simulink model "callGAMS"  (R2021b)
settings: Solver=ode1  StartTime=0.0  StopTime=20  FixedStep=1e-4  RelTol=1e-3
model workspace (MAT data in the model file):
  firstOrder = 60
  g2Max = 0
  runTime = 4
undefined symbols (not defined in the file or in its folder): c0, c1, D11, Delta, fg, G2gen, G3gen, G5gen, G6gen, G7gen, Iovc, l0, l1, Newton, r0, r1, Raphson, Rtpu, S1non, S2non, S3non, S5non, S6non, S7non, sigbuilder_block, tonvsc, Ts, Vhv, Vmv, w_pll, wc1, wdc1, wpq1, wsw1, Xtpu
libraries: simulink_extras x122, simulink x73, spsFirstOrderFilterLib x72, spsGroundLib x61, spsCurrentMeasurementLib x33, spsVoltageMeasurementLib x33, eeTransforms x24, spsabctoAlphaBetaZeroLib x12, spsControlledVoltageSourceLib x12, spsControlledCurrentSourceLib x12, spsPower3phPhasorLib x11, spsLoadFlowBusLib x9
(part 2 of 16)

== system callGAMS/sm_computation/G2 ==
  Bus Selector : BusSelector  OutputSignals=Pabc,Qabc,vqp,vdp,vqn,vdn,iqp,idp,iqn,idn,f
  Constant1 : Constant  Value=5e6
  G2 setpoint : Subsystem
  Goto1 : Goto  Commented=on  GotoTag=Pg2  TagVisibility=global
  Goto3 : Goto  Commented=on  GotoTag=vdqpng2  TagVisibility=global
  Goto4 : Goto  Commented=on  GotoTag=idqpng2  TagVisibility=global
  Goto5 : Goto  Commented=on  GotoTag=Qg2  TagVisibility=global
  Mux2 : Mux
  Mux3 : Mux
  VSC v2 : Subsystem  mask{vscmod=Phasor I-ref, fg=fg, Vhv=Vhv, Vmv=Vmv, Pconv=S2non, Rtpu=Rtpu, Xtpu=Xtpu, qmode=Active power, dmode=Reactive power, wsw=wsw1, wn_pll=w_pll, wc=wc1, wpq=wpq1, wdc=wdc1, koc=Iovc, Cdc=3100e-6, tfilt=1*(1/wsw1), negseq_en=off, fdroop_en=on, Vacdroop_en=off, LVRT_en=off, Kfdroop=0.05, fdroop_per=10, Kvdroop=0.1, Vacdroop_per=10, Vlvrt0=0.9, Vlvrt_min=0.5, Qmax_lvrt=0.9, V0pu=0.99605, theta0=-30.4161, P0=S2non*G2gen, Q0=5e6}
      mask prompts: vscmod "VSC Model"; fg "AC grid frequency (Hz)"; Vhv "Grid-side voltage (V)(LL-rms)"; Vmv "Converter-side voltage (V)(LL-rms)"; Pconv "Converter nominal power (VA)"; Rtpu "Resistance seen by the converter (p.u)"; Xtpu "Reactance seen by the converter (p.u)"; qmode "q-axis control mode"; dmode "d-axis control mode"; wsw "Switching frequency (rad/s)"; wn_pll "PLL filter natural frequency"; wc "Current-control bandwidth (rad/s)"; wpq "PQ control bandwidth (rad/s)"; wdc "DC Voltage control bandwidth(rad/s)"; koc "Overcurrent factor (p.u)"; Cdc "DC-side total capacitance (F)"; tfilt "Vabc filter time constant (s)"; negseq_en "Enable negative sequence control"; fdroop_en "Enable frequency droop"; Vacdroop_en "Enable AC voltage droop"; LVRT_en "Enable LVRT"; Kfdroop "Frequency droop (p.u)"; fdroop_per "Percentage of converter power to contribute with droop (%)"; Kvdroop "Voltage droop (p.u)"; Vacdroop_per "Percentage of converter power to contribute with droop (%)"; Vlvrt0 "initial voltage (p.u)"; Vlvrt_min "minimum voltage (p.u)"; Qmax_lvrt "max power injected at min voltage (p.u)"; V0pu "Initial terminal voltage magnitude (pu)"; theta0 "Initial terminal voltage angle (deg)"; P0 "Initial active power (W)"; Q0 "Initial reactive power (VAr)"
      mask init:
      | %% ----------------------VSC Parameters-------------------------- %%
      | j = 1i;
      | r = Vhv/Vmv;                    % Transformer ratio
      | Vmvpk = Vmv*sqrt(2)/sqrt(3);    % Converter-side voltage phase-to-ground peak-to-peak
      | Vhvpk = Vhv*sqrt(2)/sqrt(3);    % Grid-side voltage phase-to-ground peak-to-peak  
      | Vdc = 2*Vhvpk;                  % Nominal DC voltage 
      | ksw = round(wsw/(2*pi*fg));      % Calculates switching ratio
      | Iconvbase = 2*Pconv/(3*Vmvpk);  % Converter base current (A)
      | Zbmv = Vmv^2/Pconv;             % Base voltage referred to the converter side
      | Imax = koc*Iconvbase;   % Converter maximum output current
      | %Cdc = 2*Hvsc*Pconv/Vdc^2;       % DC capacitor
      | 
      | Xt = Xtpu*Zbmv;        % p.u to (Ohms)
      | Lt = Xt/(2*pi*fg);              % p.u to (H)
      | Rt = Rtpu*Zbmv;        % p.u. to (Ohms)
      | 
      | % -------------LVRT--------------%
      | Klvrt = Qmax_lvrt/(Vlvrt_min-Vlvrt0); % Defines LVRT inclination of the V/I LVRT characteristic
      | 
      | % ------------ PLL ------------- %
      | zeta_pll = 1/sqrt(2);           % Damping
      | kp_pll = 2*zeta_pll*wn_pll/(Vmvpk);
      | tau_pll = 2*zeta_pll/wn_pll;
      | 
      | % ------------ Inner-loop (current control) ------------ %
      | kp_c = Lt*wc; 
      | ti_c = Lt/Rt;
      | 
      | % -------- Outer-loop (voltage and/or power control)
      | % --- PQ closed-loop control ----
      | ti_pq = 1/wc;
      | kp_pq = 2/3*ti_pq*wpq*1/Vmvpk;
      | 
      | % --- Vdc control ----
      | damp_dc = 1/sqrt(2);
      | kp_dc = 2*Cdc*damp_dc*wdc; 
      | ki_dc = Cdc*wdc^2;
      | 
      | %% ---------------------Mask operations----------------------------%%
      | 
      | % If the box is unchecked, we set the bias value to zero
      | if ~fdroop_en; end
      | if ~Vacdroop_en; end
      | if ~LVRT_en; Klvrt = 0;  end
      | 
      | %% -------------------- Variant Subsystem ----------------------- %%
      | choice = get_param(gcb,'vscmod'); % Get choice from list
      | VSS_model = [gcb, '/VSC Model'];  % VSC electrical Model
      | VSS_meas = [gcb, '/VSC Control/Measurements']; % Measurements (PLL, Park transformation, etc)
      | VSS_mod = [gcb, '/VSC Control/Modulation']; % Modulation or reference voltage/current generation
      | VSS_ctr = [gcb, '/VSC Control/Control loops']; % Modulation or reference voltage/current generation
      | 
      | 
      | if strcmp(choice,'EMT Switching')
      |     set_param(VSS_model, 'LabelModeActiveChoice', 'EMT_SW');
      |     set_param(VSS_meas, 'LabelModeActiveChoice', 'EMT');
      |     set_param(VSS_mod, 'LabelModeActiveChoice', 'EMT_SW');
      |     set_param(VSS_ctr, 'LabelModeActiveChoice', 'EMT_and_QEMT');
      |     
      | elseif strcmp(choice,'EMT Average')
      |     set_param(VSS_model, 'LabelModeActiveChoice', 'EMT_AVG');
      |     set_param(VSS_meas, 'LabelModeActiveChoice', 'EMT');
      |     set_param(VSS_mod, 'LabelModeActiveChoice', 'EMT_AVG');
      |     set_param(VSS_ctr, 'LabelModeActiveChoice', 'EMT_and_QEMT');
      |     %set_param([VSS_meas '/EMT/Vabc filter'],'Commented','through')
      |     tfilt = 0; % No filtering in Average model
      |     
      | elseif strcmp(choice,'Phasor Quasi-EMT')
      |     set_param(VSS_model, 'LabelModeActiveChoice', 'Phasor');
      |     set_param(VSS_meas, 'LabelModeActiveChoice', 'Phasor');
      |     set_param(VSS_mod, 'LabelModeActiveChoice', 'Phasor_QEMT');
      |     set_param(VSS_ctr, 'LabelModeActiveChoice', 'EMT_and_QEMT');
      |     
      | elseif strcmp(choice,'Phasor I-1st')
      |     set_param(VSS_model, 'LabelModeActiveChoice', 'Phasor');
      |     set_param(VSS_meas, 'LabelModeActiveChoice', 'Phasor');
      |     set_param(VSS_mod, 'LabelModeActiveChoice', 'Phasor_I_and_PQ');
      |     set_param(VSS_ctr, 'LabelModeActiveChoice', 'Phasor_I_1st');
      |     
      | elseif strcmp(choice,'Phasor I-ref')
      |     set_param(VSS_model, 'LabelModeActiveChoice', 'Phasor');
      | 	set_param(VSS_meas, 'LabelModeActiveChoice', 'Phasor');
      |     set_param(VSS_mod, 'LabelModeActiveChoice', 'Phasor_I_and_PQ');
      |     set_param(VSS_ctr, 'LabelModeActiveChoice', 'Phasor_I_ref');
      |     
      | elseif strcmp(choice,'Phasor PQ-1st')
      |     set_param(VSS_model, 'LabelModeActiveChoice', 'Phasor');
      |     set_param(VSS_meas, 'LabelModeActiveChoice', 'Phasor');
      |     set_param(VSS_mod, 'LabelModeActiveChoice', 'Phasor_I_and_PQ');
      |     set_param(VSS_ctr, 'LabelModeActiveChoice', 'Phasor_PQ');
      | end
      | 
      | 
      | %% ------------------------- Converter initialization -----------------------------
      | 
      | %-------------- Electrical part ----------------------
      | theta0 = theta0*pi/180; % deg to rad
      | 
      | Vgmag = V0pu*Vhv/sqrt(3); % Phase Voltage magnitude (LG,RMS)
      | Xt = Xtpu*Zbmv; % Converting the reactance the converter sees to Ohms
      | 
      | % Grid voltage in rectangular format, with reference to the MV-side (divided by the transformer relation)
      | [Vgr,Vgi] = pol2cart(theta0,Vgmag/r);
      | Vg = complex(Vgr,Vgi);
      | 
      | % Complex power
      | S0 = complex(P0,Q0);
      | 
      | % Converter output current (RMS), with reference to the MV side
      | Ic = conj(S0/(3*Vg));
      | 
      | % Converter internal voltage (LG,RMS), with reference to the MV side
      | Vc = Vg + Ic*(Rt + j*Xt);
      | 
      | %------------------- Converter part ----------------
      | 
      | % ---------- PLL -----------
      | % The angle used in dq transformation is different in EMT and in Phasor
      | if (strcmp(choice,'EMT Switching') || strcmp(choice,'EMT Average'))
      |     thetaPLL = pi + theta0;
      | elseif (strcmp(choice,'Phasor Quasi-EMT') || strcmp(choice,'Phasor I-1st') || strcmp(choice,'Phasor I-ref') || strcmp(choice,'Phasor PQ-1st'))
      |     thetaPLL = pi;
      | end
      | 
      | 
      | % ------ dq variables --------
      | 
      | Vgq = imag(Vg*sqrt(2)*exp(-j*(thetaPLL + pi/2))); 
      | Vgd = real(Vg*sqrt(2)*exp(-j*(thetaPLL + pi/2))); 
      | 
      | Vcq = imag(Vc*sqrt(2)*exp(-j*(thetaPLL + pi/2))); 
      | Vcd = real(Vc*sqrt(2)*exp(-j*(thetaPLL + pi/2))); 
      | 
      | Icq = imag(Ic*sqrt(2)*exp(-j*(thetaPLL + pi/2))); 
      | Icd = real(Ic*sqrt(2)*exp(-j*(thetaPLL + pi/2))); 
      | 
      | % ------ Inner loop ------
      | % Now that we know the reference voltage in dq (Vc,qd), the grid voltage in dq (Vg,qd) and the converter
      | % current in dq (Ic,dq), we can calculate the PI controller output in t=0
      | % As we assume zero steady-state error, the proportional part is zero and we calculate only the integrator part (Tc,qd)
      | Tcq = Vcq - Vgq - Xt*Icd;
      | Tcd = Vcd - Vgd + Xt*Icq;
      | 
      | % ------- Outer loop -------
      | % As we know the converter current, and we know that the proportional part is zero, we calculate the
      | % integrator part (To,qd)
      | Toq = Icq;
      | Tod = Icd;
      mask TypeOptions vscmod: EMT Switching | EMT Average | Phasor Quasi-EMT | Phasor I-1st | Phasor I-ref | Phasor PQ-1st
      mask Callback vscmod:
      | % Control parameter visiblity
      | 
      | % Get the value of the Enable Bias checkbox
      | % unchecked = 'off'
      | % checked = 'on'
      | 
      | maskObj = Simulink.Mask.get(gcb);
      | 
      | wn_pll = 'on';
      | wsw = 'on';
      | DC_en = 'off';
      | 
      | vscmod = get_param(gcb,'vscmod');
      |     if strcmp(vscmod,'EMT Switching')
      |       wn_pll = 'on';
      |       wsw = 'on';
      |       tfilt = 'on';
      |     elseif strcmp(vscmod,'EMT Average')
      |         wn_pll = 'on';
      |         wsw = 'off';
      |         tfilt = 'off';
      |     elseif strcmp(vscmod,'Phasor Quasi-EMT')
      |         wn_pll = 'off';
      |         wsw = 'off';
      |         tfilt = 'off';
      |     elseif strcmp(vscmod,'Phasor I-1st')
      |         wn_pll = 'off';
      |         wsw = 'off';
      |         tfilt = 'off';
      |     elseif strcmp(vscmod,'Phasor I-ref')
      |         wn_pll = 'off';
      |         wsw = 'off';
      |         tfilt = 'off';
      |     elseif strcmp(vscmod,'Phasor PQ-1st')
      |         wn_pll = 'off';
      |         wsw = 'off';
      |         tfilt = 'off';
      |     end
      | 
      | fdroop_en = get_param(gcb,'fdroop_en');
      | Vacdroop_en = get_param(gcb,'Vacdroop_en');
      | LVRT_en = get_param(gcb,'LVRT_en');
      | negseq_en = get_param(gcb,'negseq_en');
      | qmode_str = get_param(gcb,'qmode');
      | 
      | 
      | if strcmp(qmode_str,'DC voltage')
      |     DC_en = 'on';
      | else
      |     DC_en = 'off';
      | end
      | 
      | % Set the 'MaskVisibilities' property for each parameters
      |     set_param(gcb,'MaskVisibilities',{'on','on','on','on','on','on','on','on','on',wsw,wn_pll,'on','on','on','on',DC_en,tfilt,'on','on','on','on',fdroop_en,fdroop_en,Vacdroop_en,Vacdroop_en,'on','on','on','on','on','on','on'});
      | 
      | % Make LVRT area visible when it is enabled
      | if strcmp(LVRT_en,'on')
      |   maskObj.getDialogControl('Container_LVRT').Visible = 'on';
      | else
      |     maskObj.getDialogControl('Container_LVRT').Visible = 'off';
      | end
      | 
      | % Note that the value of the bias is not handled here.
      | % See the Initialization tab
      mask TypeOptions qmode: Active power | DC voltage
      mask Callback qmode:
      | % Control parameter visiblity
      | 
      | % Get the value of the Enable Bias checkbox
      | % unchecked = 'off'
      | % checked = 'on'
      | 
      | maskObj = Simulink.Mask.get(gcb);
      | 
      | wn_pll = 'on';
      | wsw = 'on';
      | DC_en = 'off';
      | 
      | vscmod = get_param(gcb,'vscmod');
      |     if strcmp(vscmod,'EMT Switching')
      |       wn_pll = 'on';
      |       wsw = 'on';
      |       tfilt = 'on';
      |     elseif strcmp(vscmod,'EMT Average')
      |         wn_pll = 'on';
      |         wsw = 'off';
      |         tfilt = 'off';
      |     elseif strcmp(vscmod,'Phasor Quasi-EMT')
      |         wn_pll = 'off';
      |         wsw = 'off';
      |         tfilt = 'off';
      |     elseif strcmp(vscmod,'Phasor I-1st')
      |         wn_pll = 'off';
      |         wsw = 'off';
      |         tfilt = 'off';
      |     elseif strcmp(vscmod,'Phasor I-ref')
      |         wn_pll = 'off';
      |         wsw = 'off';
      |         tfilt = 'off';
      |     elseif strcmp(vscmod,'Phasor PQ-1st')
      |         wn_pll = 'off';
      |         wsw = 'off';
      |         tfilt = 'off';
      |     end
      | 
      | fdroop_en = get_param(gcb,'fdroop_en');
      | Vacdroop_en = get_param(gcb,'Vacdroop_en');
      | LVRT_en = get_param(gcb,'LVRT_en');
      | negseq_en = get_param(gcb,'negseq_en');
      | qmode_str = get_param(gcb,'qmode');
      | 
      | 
      | if strcmp(qmode_str,'DC voltage')
      |     DC_en = 'on';
      | else
      |     DC_en = 'off';
      | end
      | 
      | % Set the 'MaskVisibilities' property for each parameters
      |     set_param(gcb,'MaskVisibilities',{'on','on','on','on','on','on','on','on','on',wsw,wn_pll,'on','on','on','on',DC_en,tfilt,'on','on','on','on',fdroop_en,fdroop_en,Vacdroop_en,Vacdroop_en,'on','on','on','on','on','on','on'});
      | 
      | % Make LVRT area visible when it is enabled
      | if strcmp(LVRT_en,'on')
      |   maskObj.getDialogControl('Container_LVRT').Visible = 'on';
      | else
      |     maskObj.getDialogControl('Container_LVRT').Visible = 'off';
      | end
      | 
      | % Note that the value of the bias is not handled here.
      | % See the Initialization tab
      mask TypeOptions dmode: Reactive power | AC voltage
      mask Callback fdroop_en:
      | % Control parameter visiblity
      | 
      | % Get the value of the Enable Bias checkbox
      | % unchecked = 'off'
      | % checked = 'on'
      | 
      | maskObj = Simulink.Mask.get(gcb);
      | 
      | wn_pll = 'on';
      | wsw = 'on';
      | DC_en = 'off';
      | 
      | vscmod = get_param(gcb,'vscmod');
      |     if strcmp(vscmod,'EMT Switching')
      |       wn_pll = 'on';
      |       wsw = 'on';
      |       tfilt = 'on';
      |     elseif strcmp(vscmod,'EMT Average')
      |         wn_pll = 'on';
      |         wsw = 'off';
      |         tfilt = 'off';
      |     elseif strcmp(vscmod,'Phasor Quasi-EMT')
      |         wn_pll = 'off';
      |         wsw = 'off';
      |         tfilt = 'off';
      |     elseif strcmp(vscmod,'Phasor I-1st')
      |         wn_pll = 'off';
      |         wsw = 'off';
      |         tfilt = 'off';
      |     elseif strcmp(vscmod,'Phasor I-ref')
      |         wn_pll = 'off';
      |         wsw = 'off';
      |         tfilt = 'off';
      |     elseif strcmp(vscmod,'Phasor PQ-1st')
      |         wn_pll = 'off';
      |         wsw = 'off';
      |         tfilt = 'off';
      |     end
      | 
      | fdroop_en = get_param(gcb,'fdroop_en');
      | Vacdroop_en = get_param(gcb,'Vacdroop_en');
      | LVRT_en = get_param(gcb,'LVRT_en');
      | negseq_en = get_param(gcb,'negseq_en');
      | qmode_str = get_param(gcb,'qmode');
      | 
      | 
      | if strcmp(qmode_str,'DC voltage')
      |     DC_en = 'on';
      | else
      |     DC_en = 'off';
      | end
      | 
      | % Set the 'MaskVisibilities' property for each parameters
      |     set_param(gcb,'MaskVisibilities',{'on','on','on','on','on','on','on','on','on',wsw,wn_pll,'on','on','on','on',DC_en,tfilt,'on','on','on','on',fdroop_en,fdroop_en,Vacdroop_en,Vacdroop_en,'on','on','on','on','on','on','on'});
      | 
      | % Make LVRT area visible when it is enabled
      | if strcmp(LVRT_en,'on')
      |   maskObj.getDialogControl('Container_LVRT').Visible = 'on';
      | else
      |     maskObj.getDialogControl('Container_LVRT').Visible = 'off';
      | end
      | 
      | % Note that the value of the bias is not handled here.
      | % See the Initialization tab
      mask Callback Vacdroop_en:
      | % Control parameter visiblity
      | 
      | % Get the value of the Enable Bias checkbox
      | % unchecked = 'off'
      | % checked = 'on'
      | 
      | maskObj = Simulink.Mask.get(gcb);
      | 
      | wn_pll = 'on';
      | wsw = 'on';
      | DC_en = 'off';
      | 
      | vscmod = get_param(gcb,'vscmod');
      |     if strcmp(vscmod,'EMT Switching')
      |       wn_pll = 'on';
      |       wsw = 'on';
      |       tfilt = 'on';
      |     elseif strcmp(vscmod,'EMT Average')
      |         wn_pll = 'on';
      |         wsw = 'off';
      |         tfilt = 'off';
      |     elseif strcmp(vscmod,'Phasor Quasi-EMT')
      |         wn_pll = 'off';
      |         wsw = 'off';
      |         tfilt = 'off';
      |     elseif strcmp(vscmod,'Phasor I-1st')
      |         wn_pll = 'off';
      |         wsw = 'off';
      |         tfilt = 'off';
      |     elseif strcmp(vscmod,'Phasor I-ref')
      |         wn_pll = 'off';
      |         wsw = 'off';
      |         tfilt = 'off';
      |     elseif strcmp(vscmod,'Phasor PQ-1st')
      |         wn_pll = 'off';
      |         wsw = 'off';
      |         tfilt = 'off';
      |     end
      | 
      | fdroop_en = get_param(gcb,'fdroop_en');
      | Vacdroop_en = get_param(gcb,'Vacdroop_en');
      | LVRT_en = get_param(gcb,'LVRT_en');
      | negseq_en = get_param(gcb,'negseq_en');
      | qmode_str = get_param(gcb,'qmode');
      | 
      | 
      | if strcmp(qmode_str,'DC voltage')
      |     DC_en = 'on';
      | else
      |     DC_en = 'off';
      | end
      | 
      | % Set the 'MaskVisibilities' property for each parameters
      |     set_param(gcb,'MaskVisibilities',{'on','on','on','on','on','on','on','on','on',wsw,wn_pll,'on','on','on','on',DC_en,tfilt,'on','on','on','on',fdroop_en,fdroop_en,Vacdroop_en,Vacdroop_en,'on','on','on','on','on','on','on'});
      | 
      | % Make LVRT area visible when it is enabled
      | if strcmp(LVRT_en,'on')
      |   maskObj.getDialogControl('Container_LVRT').Visible = 'on';
      | else
      |     maskObj.getDialogControl('Container_LVRT').Visible = 'off';
      | end
      | 
      | % Note that the value of the bias is not handled here.
      | % See the Initialization tab
      mask Callback LVRT_en:
      | % Control parameter visiblity
      | 
      | % Get the value of the Enable Bias checkbox
      | % unchecked = 'off'
      | % checked = 'on'
      | 
      | maskObj = Simulink.Mask.get(gcb);
      | 
      | wn_pll = 'on';
      | wsw = 'on';
      | DC_en = 'off';
      | 
      | vscmod = get_param(gcb,'vscmod');
      |     if strcmp(vscmod,'EMT Switching')
      |       wn_pll = 'on';
      |       wsw = 'on';
      |       tfilt = 'on';
      |     elseif strcmp(vscmod,'EMT Average')
      |         wn_pll = 'on';
      |         wsw = 'off';
      |         tfilt = 'off';
      |     elseif strcmp(vscmod,'Phasor Quasi-EMT')
      |         wn_pll = 'off';
      |         wsw = 'off';
      |         tfilt = 'off';
      |     elseif strcmp(vscmod,'Phasor I-1st')
      |         wn_pll = 'off';
      |         wsw = 'off';
      |         tfilt = 'off';
      |     elseif strcmp(vscmod,'Phasor I-ref')
      |         wn_pll = 'off';
      |         wsw = 'off';
      |         tfilt = 'off';
      |     elseif strcmp(vscmod,'Phasor PQ-1st')
      |         wn_pll = 'off';
      |         wsw = 'off';
      |         tfilt = 'off';
      |     end
      | 
      | fdroop_en = get_param(gcb,'fdroop_en');
      | Vacdroop_en = get_param(gcb,'Vacdroop_en');
      | LVRT_en = get_param(gcb,'LVRT_en');
      | negseq_en = get_param(gcb,'negseq_en');
      | qmode_str = get_param(gcb,'qmode');
      | 
      | 
      | if strcmp(qmode_str,'DC voltage')
      |     DC_en = 'on';
      | else
      |     DC_en = 'off';
      | end
      | 
      | % Set the 'MaskVisibilities' property for each parameters
      |     set_param(gcb,'MaskVisibilities',{'on','on','on','on','on','on','on','on','on',wsw,wn_pll,'on','on','on','on',DC_en,tfilt,'on','on','on','on',fdroop_en,fdroop_en,Vacdroop_en,Vacdroop_en,'on','on','on','on','on','on','on'});
      | 
      | % Make LVRT area visible when it is enabled
      | if strcmp(LVRT_en,'on')
      |   maskObj.getDialogControl('Container_LVRT').Visible = 'on';
      | else
      |     maskObj.getDialogControl('Container_LVRT').Visible = 'off';
      | end
      | 
      | % Note that the value of the bias is not handled here.
      | % See the Initialization tab
      mask DialogControl DescTextVar Prompt: -------------------------------------Three-phase VSC model---------------------------------------
      mask DialogControl Tab1 Prompt: Electrical parameters
      mask DialogControl Tab2 Prompt: Control parameters
      mask DialogControl Tab3 Prompt: Other parameters
      mask DialogControl Container_LVRT Prompt: LVRT
      mask DialogControl Tab4 Prompt: Power flow
      mask Display:
      | choice = get_param(gcb,'vscmod');
      | if strcmp(choice,'Phasor Quasi-EMT')
      |     disp('VSC\n\n')
      |     disp('\n\nPhasor\n\n')
      |     disp('\n\nQuasi-EMT')
      | elseif strcmp(choice,'EMT Average')
      |     disp('VSC\n')
      |     disp('\nEMT AVG')
      | elseif strcmp(choice,'EMT Switching')
      |     disp('VSC\n')
      |     disp('\nEMT SW')
      | elseif strcmp(choice,'Phasor I-1st')
      |     disp('VSC\n\n')
      |     disp('\n\nPhasor\n\n')
      |     disp('\n\nI 1st')
      | elseif strcmp(choice,'Phasor I-ref')
      |     disp('VSC\n\n')
      |     disp('\n\nPhasor\n\n')
      |     disp('\n\nI ref')
      | elseif strcmp(choice,'Phasor PQ-1st')
      |     disp('VSC\n\n')
      |     disp('\n\nPhasor\n\n')
      |     disp('\n\nPQ 1st')
      | end
  A : PMIOPort  Side=Right
  B : PMIOPort  Port=2  Side=Right
  C : PMIOPort  Port=3  Side=Right
  Output : Outport  VectorParamsAs1DForOutWhenUnconnected=off
  tag scope: fg2=global
  wires:
  Bus Selector/9 -> Mux3/3  "<iqn>"
  Bus Selector/3 -> Mux2/1  "<vqp>"
  Bus Selector/4 -> Mux2/2  "<vdp>"
  Bus Selector/8 -> Mux3/2  "<idp>"
  Mux3/1 -> Goto4/1
  Bus Selector/10 -> Mux3/4  "<idn>"
  Mux2/1 -> Goto3/1
  Bus Selector/6 -> Mux2/4  "<vdn>"
  Bus Selector/7 -> Mux3/1  "<iqp>"
  VSC v2/1(m) -> Bus Selector/1
  Bus Selector/5 -> Mux2/3  "<vqn>"
  Bus Selector/11 -> [fg2]  "<f>"
  Bus Selector/1 -> Goto1/1  "<Pabc>"
  Bus Selector/2 -> Goto5/1  "<Qabc>"
  Constant1/1 -> VSC v2/2(Qset)
  G2 setpoint/1(Out1) -> Output/1, VSC v2/1(Pset)
  connections:
  VSC v2/LConn2 -- B/RConn1
  VSC v2/LConn1 -- A/RConn1
  VSC v2/LConn3 -- C/RConn1

== system callGAMS/sm_computation/G3 ==
  Bus Selector : BusSelector  OutputSignals=Pabc,Qabc,vqp,vdp,vqn,vdn,iqp,idp,iqn,idn,f
  Constant1 : Constant  Value=5e6
  G3 setpoint : Subsystem
  Goto1 : Goto  Commented=on  GotoTag=Pg3  TagVisibility=global
  Goto3 : Goto  Commented=on  GotoTag=vdqpng3  TagVisibility=global
  Goto4 : Goto  Commented=on  GotoTag=idqpng3  TagVisibility=global
  Goto5 : Goto  Commented=on  GotoTag=Qg3  TagVisibility=global
  Mux2 : Mux
  Mux3 : Mux
  VSC v2 : Subsystem  mask{vscmod=Phasor I-ref, fg=fg, Vhv=Vhv, Vmv=Vmv, Pconv=S3non, Rtpu=Rtpu, Xtpu=Xtpu, qmode=Active power, dmode=Reactive power, wsw=wsw1, wn_pll=w_pll, wc=wc1, wpq=wpq1, wdc=wdc1, koc=Iovc, Cdc=3100e-6, tfilt=1*(1/wsw1), negseq_en=off, fdroop_en=on, Vacdroop_en=off, LVRT_en=off, Kfdroop=0.05, fdroop_per=10, Kvdroop=0.1, Vacdroop_per=10, Vlvrt0=0.9, Vlvrt_min=0.5, Qmax_lvrt=0.9, V0pu=0.99447, theta0=-30.6528, P0=S3non*G3gen, Q0=5e6}
      mask prompts: vscmod "VSC Model"; fg "AC grid frequency (Hz)"; Vhv "Grid-side voltage (V)(LL-rms)"; Vmv "Converter-side voltage (V)(LL-rms)"; Pconv "Converter nominal power (VA)"; Rtpu "Resistance seen by the converter (p.u)"; Xtpu "Reactance seen by the converter (p.u)"; qmode "q-axis control mode"; dmode "d-axis control mode"; wsw "Switching frequency (rad/s)"; wn_pll "PLL filter natural frequency"; wc "Current-control bandwidth (rad/s)"; wpq "PQ control bandwidth (rad/s)"; wdc "DC Voltage control bandwidth(rad/s)"; koc "Overcurrent factor (p.u)"; Cdc "DC-side total capacitance (F)"; tfilt "Vabc filter time constant (s)"; negseq_en "Enable negative sequence control"; fdroop_en "Enable frequency droop"; Vacdroop_en "Enable AC voltage droop"; LVRT_en "Enable LVRT"; Kfdroop "Frequency droop (p.u)"; fdroop_per "Percentage of converter power to contribute with droop (%)"; Kvdroop "Voltage droop (p.u)"; Vacdroop_per "Percentage of converter power to contribute with droop (%)"; Vlvrt0 "initial voltage (p.u)"; Vlvrt_min "minimum voltage (p.u)"; Qmax_lvrt "max power injected at min voltage (p.u)"; V0pu "Initial terminal voltage magnitude (pu)"; theta0 "Initial terminal voltage angle (deg)"; P0 "Initial active power (W)"; Q0 "Initial reactive power (VAr)"
      mask init: same as callGAMS/sm_computation/G2/VSC v2
      mask TypeOptions vscmod: EMT Switching | EMT Average | Phasor Quasi-EMT | Phasor I-1st | Phasor I-ref | Phasor PQ-1st
      mask Callback vscmod:
      | % Control parameter visiblity
      | 
      | % Get the value of the Enable Bias checkbox
      | % unchecked = 'off'
      | % checked = 'on'
      | 
      | maskObj = Simulink.Mask.get(gcb);
      | 
      | wn_pll = 'on';
      | wsw = 'on';
      | DC_en = 'off';
      | 
      | vscmod = get_param(gcb,'vscmod');
      |     if strcmp(vscmod,'EMT Switching')
      |       wn_pll = 'on';
      |       wsw = 'on';
      |       tfilt = 'on';
      |     elseif strcmp(vscmod,'EMT Average')
      |         wn_pll = 'on';
      |         wsw = 'off';
      |         tfilt = 'off';
      |     elseif strcmp(vscmod,'Phasor Quasi-EMT')
      |         wn_pll = 'off';
      |         wsw = 'off';
      |         tfilt = 'off';
      |     elseif strcmp(vscmod,'Phasor I-1st')
      |         wn_pll = 'off';
      |         wsw = 'off';
      |         tfilt = 'off';
      |     elseif strcmp(vscmod,'Phasor I-ref')
      |         wn_pll = 'off';
      |         wsw = 'off';
      |         tfilt = 'off';
      |     elseif strcmp(vscmod,'Phasor PQ-1st')
      |         wn_pll = 'off';
      |         wsw = 'off';
      |         tfilt = 'off';
      |     end
      | 
      | fdroop_en = get_param(gcb,'fdroop_en');
      | Vacdroop_en = get_param(gcb,'Vacdroop_en');
      | LVRT_en = get_param(gcb,'LVRT_en');
      | negseq_en = get_param(gcb,'negseq_en');
      | qmode_str = get_param(gcb,'qmode');
      | 
      | 
      | if strcmp(qmode_str,'DC voltage')
      |     DC_en = 'on';
      | else
      |     DC_en = 'off';
      | end
      | 
      | % Set the 'MaskVisibilities' property for each parameters
      |     set_param(gcb,'MaskVisibilities',{'on','on','on','on','on','on','on','on','on',wsw,wn_pll,'on','on','on','on',DC_en,tfilt,'on','on','on','on',fdroop_en,fdroop_en,Vacdroop_en,Vacdroop_en,'on','on','on','on','on','on','on'});
      | 
      | % Make LVRT area visible when it is enabled
      | if strcmp(LVRT_en,'on')
      |   maskObj.getDialogControl('Container_LVRT').Visible = 'on';
      | else
      |     maskObj.getDialogControl('Container_LVRT').Visible = 'off';
      | end
      | 
      | % Note that the value of the bias is not handled here.
      | % See the Initialization tab
      mask TypeOptions qmode: Active power | DC voltage
      mask Callback qmode:
      | % Control parameter visiblity
      | 
      | % Get the value of the Enable Bias checkbox
      | % unchecked = 'off'
      | % checked = 'on'
      | 
      | maskObj = Simulink.Mask.get(gcb);
      | 
      | wn_pll = 'on';
      | wsw = 'on';
      | DC_en = 'off';
      | 
      | vscmod = get_param(gcb,'vscmod');
      |     if strcmp(vscmod,'EMT Switching')
      |       wn_pll = 'on';
      |       wsw = 'on';
      |       tfilt = 'on';
      |     elseif strcmp(vscmod,'EMT Average')
      |         wn_pll = 'on';
      |         wsw = 'off';
      |         tfilt = 'off';
      |     elseif strcmp(vscmod,'Phasor Quasi-EMT')
      |         wn_pll = 'off';
      |         wsw = 'off';
      |         tfilt = 'off';
      |     elseif strcmp(vscmod,'Phasor I-1st')
      |         wn_pll = 'off';
      |         wsw = 'off';
      |         tfilt = 'off';
      |     elseif strcmp(vscmod,'Phasor I-ref')
      |         wn_pll = 'off';
      |         wsw = 'off';
      |         tfilt = 'off';
      |     elseif strcmp(vscmod,'Phasor PQ-1st')
      |         wn_pll = 'off';
      |         wsw = 'off';
      |         tfilt = 'off';
      |     end
      | 
      | fdroop_en = get_param(gcb,'fdroop_en');
      | Vacdroop_en = get_param(gcb,'Vacdroop_en');
      | LVRT_en = get_param(gcb,'LVRT_en');
      | negseq_en = get_param(gcb,'negseq_en');
      | qmode_str = get_param(gcb,'qmode');
      | 
      | 
      | if strcmp(qmode_str,'DC voltage')
      |     DC_en = 'on';
      | else
      |     DC_en = 'off';
      | end
      | 
      | % Set the 'MaskVisibilities' property for each parameters
      |     set_param(gcb,'MaskVisibilities',{'on','on','on','on','on','on','on','on','on',wsw,wn_pll,'on','on','on','on',DC_en,tfilt,'on','on','on','on',fdroop_en,fdroop_en,Vacdroop_en,Vacdroop_en,'on','on','on','on','on','on','on'});
      | 
      | % Make LVRT area visible when it is enabled
      | if strcmp(LVRT_en,'on')
      |   maskObj.getDialogControl('Container_LVRT').Visible = 'on';
      | else
      |     maskObj.getDialogControl('Container_LVRT').Visible = 'off';
      | end
      | 
      | % Note that the value of the bias is not handled here.
      | % See the Initialization tab
      mask TypeOptions dmode: Reactive power | AC voltage
      mask Callback fdroop_en:
      | % Control parameter visiblity
      | 
      | % Get the value of the Enable Bias checkbox
      | % unchecked = 'off'
      | % checked = 'on'
      | 
      | maskObj = Simulink.Mask.get(gcb);
      | 
      | wn_pll = 'on';
      | wsw = 'on';
      | DC_en = 'off';
      | 
      | vscmod = get_param(gcb,'vscmod');
      |     if strcmp(vscmod,'EMT Switching')
      |       wn_pll = 'on';
      |       wsw = 'on';
      |       tfilt = 'on';
      |     elseif strcmp(vscmod,'EMT Average')
      |         wn_pll = 'on';
      |         wsw = 'off';
      |         tfilt = 'off';
      |     elseif strcmp(vscmod,'Phasor Quasi-EMT')
      |         wn_pll = 'off';
      |         wsw = 'off';
      |         tfilt = 'off';
      |     elseif strcmp(vscmod,'Phasor I-1st')
      |         wn_pll = 'off';
      |         wsw = 'off';
      |         tfilt = 'off';
      |     elseif strcmp(vscmod,'Phasor I-ref')
      |         wn_pll = 'off';
      |         wsw = 'off';
      |         tfilt = 'off';
      |     elseif strcmp(vscmod,'Phasor PQ-1st')
      |         wn_pll = 'off';
      |         wsw = 'off';
      |         tfilt = 'off';
      |     end
      | 
      | fdroop_en = get_param(gcb,'fdroop_en');
      | Vacdroop_en = get_param(gcb,'Vacdroop_en');
      | LVRT_en = get_param(gcb,'LVRT_en');
      | negseq_en = get_param(gcb,'negseq_en');
      | qmode_str = get_param(gcb,'qmode');
      | 
      | 
      | if strcmp(qmode_str,'DC voltage')
      |     DC_en = 'on';
      | else
      |     DC_en = 'off';
      | end
      | 
      | % Set the 'MaskVisibilities' property for each parameters
      |     set_param(gcb,'MaskVisibilities',{'on','on','on','on','on','on','on','on','on',wsw,wn_pll,'on','on','on','on',DC_en,tfilt,'on','on','on','on',fdroop_en,fdroop_en,Vacdroop_en,Vacdroop_en,'on','on','on','on','on','on','on'});
      | 
      | % Make LVRT area visible when it is enabled
      | if strcmp(LVRT_en,'on')
      |   maskObj.getDialogControl('Container_LVRT').Visible = 'on';
      | else
      |     maskObj.getDialogControl('Container_LVRT').Visible = 'off';
      | end
      | 
      | % Note that the value of the bias is not handled here.
      | % See the Initialization tab
      mask Callback Vacdroop_en:
      | % Control parameter visiblity
      | 
      | % Get the value of the Enable Bias checkbox
      | % unchecked = 'off'
      | % checked = 'on'
      | 
      | maskObj = Simulink.Mask.get(gcb);
      | 
      | wn_pll = 'on';
      | wsw = 'on';
      | DC_en = 'off';
      | 
      | vscmod = get_param(gcb,'vscmod');
      |     if strcmp(vscmod,'EMT Switching')
      |       wn_pll = 'on';
      |       wsw = 'on';
      |       tfilt = 'on';
      |     elseif strcmp(vscmod,'EMT Average')
      |         wn_pll = 'on';
      |         wsw = 'off';
      |         tfilt = 'off';
      |     elseif strcmp(vscmod,'Phasor Quasi-EMT')
      |         wn_pll = 'off';
      |         wsw = 'off';
      |         tfilt = 'off';
      |     elseif strcmp(vscmod,'Phasor I-1st')
      |         wn_pll = 'off';
      |         wsw = 'off';
      |         tfilt = 'off';
      |     elseif strcmp(vscmod,'Phasor I-ref')
      |         wn_pll = 'off';
      |         wsw = 'off';
      |         tfilt = 'off';
      |     elseif strcmp(vscmod,'Phasor PQ-1st')
      |         wn_pll = 'off';
      |         wsw = 'off';
      |         tfilt = 'off';
      |     end
      | 
      | fdroop_en = get_param(gcb,'fdroop_en');
      | Vacdroop_en = get_param(gcb,'Vacdroop_en');
      | LVRT_en = get_param(gcb,'LVRT_en');
      | negseq_en = get_param(gcb,'negseq_en');
      | qmode_str = get_param(gcb,'qmode');
      | 
      | 
      | if strcmp(qmode_str,'DC voltage')
      |     DC_en = 'on';
      | else
      |     DC_en = 'off';
      | end
      | 
      | % Set the 'MaskVisibilities' property for each parameters
      |     set_param(gcb,'MaskVisibilities',{'on','on','on','on','on','on','on','on','on',wsw,wn_pll,'on','on','on','on',DC_en,tfilt,'on','on','on','on',fdroop_en,fdroop_en,Vacdroop_en,Vacdroop_en,'on','on','on','on','on','on','on'});
      | 
      | % Make LVRT area visible when it is enabled
      | if strcmp(LVRT_en,'on')
      |   maskObj.getDialogControl('Container_LVRT').Visible = 'on';
      | else
      |     maskObj.getDialogControl('Container_LVRT').Visible = 'off';
      | end
      | 
      | % Note that the value of the bias is not handled here.
      | % See the Initialization tab
      mask Callback LVRT_en:
      | % Control parameter visiblity
      | 
      | % Get the value of the Enable Bias checkbox
      | % unchecked = 'off'
      | % checked = 'on'
      | 
      | maskObj = Simulink.Mask.get(gcb);
      | 
      | wn_pll = 'on';
      | wsw = 'on';
      | DC_en = 'off';
      | 
      | vscmod = get_param(gcb,'vscmod');
      |     if strcmp(vscmod,'EMT Switching')
      |       wn_pll = 'on';
      |       wsw = 'on';
      |       tfilt = 'on';
      |     elseif strcmp(vscmod,'EMT Average')
      |         wn_pll = 'on';
      |         wsw = 'off';
      |         tfilt = 'off';
      |     elseif strcmp(vscmod,'Phasor Quasi-EMT')
      |         wn_pll = 'off';
      |         wsw = 'off';
      |         tfilt = 'off';
      |     elseif strcmp(vscmod,'Phasor I-1st')
      |         wn_pll = 'off';
      |         wsw = 'off';
      |         tfilt = 'off';
      |     elseif strcmp(vscmod,'Phasor I-ref')
      |         wn_pll = 'off';
      |         wsw = 'off';
      |         tfilt = 'off';
      |     elseif strcmp(vscmod,'Phasor PQ-1st')
      |         wn_pll = 'off';
      |         wsw = 'off';
      |         tfilt = 'off';
      |     end
      | 
      | fdroop_en = get_param(gcb,'fdroop_en');
      | Vacdroop_en = get_param(gcb,'Vacdroop_en');
      | LVRT_en = get_param(gcb,'LVRT_en');
      | negseq_en = get_param(gcb,'negseq_en');
      | qmode_str = get_param(gcb,'qmode');
      | 
      | 
      | if strcmp(qmode_str,'DC voltage')
      |     DC_en = 'on';
      | else
      |     DC_en = 'off';
      | end
      | 
      | % Set the 'MaskVisibilities' property for each parameters
      |     set_param(gcb,'MaskVisibilities',{'on','on','on','on','on','on','on','on','on',wsw,wn_pll,'on','on','on','on',DC_en,tfilt,'on','on','on','on',fdroop_en,fdroop_en,Vacdroop_en,Vacdroop_en,'on','on','on','on','on','on','on'});
      | 
      | % Make LVRT area visible when it is enabled
      | if strcmp(LVRT_en,'on')
      |   maskObj.getDialogControl('Container_LVRT').Visible = 'on';
      | else
      |     maskObj.getDialogControl('Container_LVRT').Visible = 'off';
      | end
      | 
      | % Note that the value of the bias is not handled here.
      | % See the Initialization tab
      mask DialogControl DescTextVar Prompt: -------------------------------------Three-phase VSC model---------------------------------------
      mask DialogControl Tab1 Prompt: Electrical parameters
      mask DialogControl Tab2 Prompt: Control parameters
      mask DialogControl Tab3 Prompt: Other parameters
      mask DialogControl Container_LVRT Prompt: LVRT
      mask DialogControl Tab4 Prompt: Power flow
      mask Display:
      | choice = get_param(gcb,'vscmod');
      | if strcmp(choice,'Phasor Quasi-EMT')
      |     disp('VSC\n\n')
      |     disp('\n\nPhasor\n\n')
      |     disp('\n\nQuasi-EMT')
      | elseif strcmp(choice,'EMT Average')
      |     disp('VSC\n')
      |     disp('\nEMT AVG')
      | elseif strcmp(choice,'EMT Switching')
      |     disp('VSC\n')
      |     disp('\nEMT SW')
      | elseif strcmp(choice,'Phasor I-1st')
      |     disp('VSC\n\n')
      |     disp('\n\nPhasor\n\n')
      |     disp('\n\nI 1st')
      | elseif strcmp(choice,'Phasor I-ref')
      |     disp('VSC\n\n')
      |     disp('\n\nPhasor\n\n')
      |     disp('\n\nI ref')
      | elseif strcmp(choice,'Phasor PQ-1st')
      |     disp('VSC\n\n')
      |     disp('\n\nPhasor\n\n')
      |     disp('\n\nPQ 1st')
      | end
  A : PMIOPort  Side=Right
  B : PMIOPort  Port=2  Side=Right
  C : PMIOPort  Port=3  Side=Right
  tag scope: fg3=global
  wires:
  Bus Selector/11 -> [fg3]  "<f>"
  Bus Selector/5 -> Mux2/3  "<vqn>"
  VSC v2/1(m) -> Bus Selector/1
  Bus Selector/7 -> Mux3/1  "<iqp>"
  Bus Selector/6 -> Mux2/4  "<vdn>"
  Mux2/1 -> Goto3/1
  Bus Selector/10 -> Mux3/4  "<idn>"
  Mux3/1 -> Goto4/1
  Bus Selector/8 -> Mux3/2  "<idp>"
  Bus Selector/1 -> Goto1/1  "<Pabc>"
  Bus Selector/4 -> Mux2/2  "<vdp>"
  Bus Selector/3 -> Mux2/1  "<vqp>"
  Bus Selector/9 -> Mux3/3  "<iqn>"
  Bus Selector/2 -> Goto5/1  "<Qabc>"
  Constant1/1 -> VSC v2/2(Qset)
  G3 setpoint/1(Out1) -> VSC v2/1(Pset)
  connections:
  VSC v2/LConn3 -- C/RConn1
  A/RConn1 -- VSC v2/LConn1
  VSC v2/LConn2 -- B/RConn1
